simulink model "simulik_DSAS"  (R2023a)
settings: Solver=FixedStepAuto  StartTime=0.0  StopTime=6000*3  FixedStep=1  RelTol=1e-3
values from neighbouring files (symbols this model uses):
  X_init_cible = [x_init(1);y_init(1);z_init(1);Vx_init(1);Vy_init(1);Vz_init(1)]    [initialisation_a_distribuer.m]
settings Model: Creator=franc  LastModifiedBy=franc
settings DataIOCC: ReturnWorkspaceOutputs=off

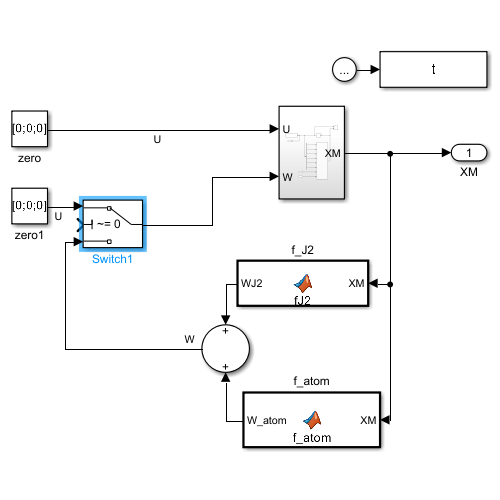
[thumbnail: Simulink's stored preview of the top-level diagram]
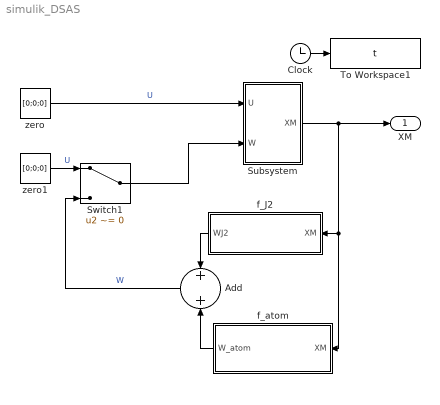
== system simulik_DSAS ==
  Add : Sum
  Clock : Clock
  Subsystem : Subsystem
  Switch1 : Switch  Criteria=u2 ~= 0  SaturateOnIntegerOverflow=off  InputSameDT=off
  To Workspace1 : ToWorkspace  VariableName=t  SampleTime=-1
  f_J2 : MATLAB Function  TreatAsAtomicUnit=on
  f_atom : MATLAB Function  TreatAsAtomicUnit=on
  zero : Constant  Value=[0;0;0]
  zero1 : Constant  Value=[0;0;0]
  XM : Outport
  wires:
  Clock/1 -> To Workspace1/1
  zero/1 -> Subsystem/1(U)  "U"
  Subsystem/1(XM) -> f_atom/1(XM), f_J2/1(XM), XM/1
  zero1/1 -> Switch1/1  "U"
  Add/1 -> Switch1/3  "W"
  Switch1/1 -> Subsystem/2(W)
  f_J2/1(WJ2) -> Add/1
  f_atom/1(W_atom) -> Add/2

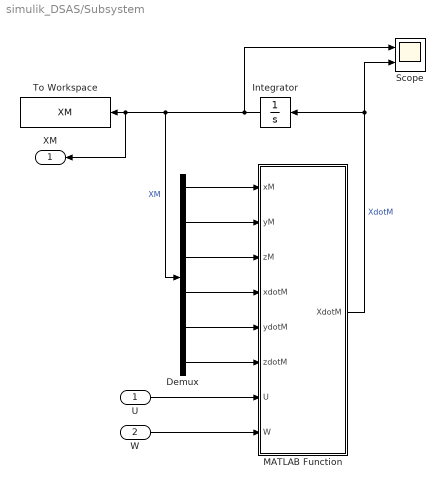
== system simulik_DSAS/Subsystem ==
  U : Inport
  W : Inport  Port=2
  Demux : Demux  Outputs=6
  Integrator : Integrator  InitialCondition=X_init_cible
  MATLAB Function : MATLAB Function  TreatAsAtomicUnit=on
  Scope : Scope  NumInputPorts=2
  To Workspace : ToWorkspace  VariableName=XM  SampleTime=-1
      settings: Save2DSignal=2-D array (concatenate along first dimension)
  XM : Outport
  wires:
  Demux/5 -> MATLAB Function/5(ydotM)
  Demux/1 -> MATLAB Function/1(xM)
  Demux/6 -> MATLAB Function/6(zdotM)
  MATLAB Function/1(XdotM) -> Scope/2, Integrator/1  "XdotM"
  Demux/4 -> MATLAB Function/4(xdotM)
  Integrator/1 -> Scope/1, Demux/1, XM/1, To Workspace/1  "XM"
  Demux/2 -> MATLAB Function/2(yM)
  Demux/3 -> MATLAB Function/3(zM)
  U/1 -> MATLAB Function/7(U)
  W/1 -> MATLAB Function/8(W)

== matlab function simulik_DSAS/Subsystem/MATLAB Function ==
  data: xM input; yM input; zM input; xdotM input; ydotM input; zdotM input; XdotM output; U input; W input
function XdotM = f(xM,yM,zM,xdotM,ydotM,zdotM, U, W)
mu = 3.986e14; 
BW = [  zeros(3,3);
        eye(3)];

BU = [  eye(3);
        zeros(3,3)];


XdotM = [   xdotM;
            ydotM;
            zdotM;
            -mu/sqrt((xM^2 + yM^2 + zM^2)^3)*xM;
            -mu/sqrt((xM^2 + yM^2 + zM^2)^3)*yM;
            -mu/sqrt((xM^2 + yM^2 + zM^2)^3)*zM] + BU*U + BW*W;

== matlab function simulik_DSAS/f_atom ==
  data: XM input; W_atom output
function W_atom = f_atom(XM)

rho_0 = 6.3e-13; 
rho = rho_0; 
S = 2; 
m = 191.1; 
CD = 2; 

W_atom = [  -rho*S*CD*sqrt(XM(4)^2+XM(5)^2+XM(6)^2)/2/m*XM(4)
            -rho*S*CD*sqrt(XM(4)^2+XM(5)^2+XM(6)^2)/2/m*XM(5)
            -rho*S*CD*sqrt(XM(4)^2+XM(5)^2+XM(6)^2)/2/m*XM(6) ];

== matlab function simulik_DSAS/f_J2 ==
  data: XM input; WJ2 output
function WJ2 = fJ2(XM)

mu = 3.986e14;          % constante gravitationnnelle 
J2 = 1.082616e-3;       % second harmonique 
Req = 6378e3;           % rayon terrestre (m)
WJ2 = 1/2*mu*J2*Req*Req*(3/sqrt(XM(1)^2+XM(2)^2+XM(3)^2)^4 - 15*XM(3)/sqrt(XM(1)^2+XM(2)^2+XM(3)^2)^6)*[XM(1);XM(2);XM(3)]/sqrt(XM(1)^2+XM(2)^2+XM(3)^2);
